simulink model "sinewave"  (R2017a)
settings: Solver=VariableStepAuto  StartTime=0.0  StopTime=100E-6  RelTol=1e-3
libraries: hdlsllib x2
settings Model: Creator=beckmanf  LastModifiedBy=beckmanf
settings OptimizationCC: BlockReduction=off  ConditionallyExecuteInputs=off  DefaultParameterBehavior=Inlined
settings DebuggingCC: AlgebraicLoopMsg=error
settings HardwareCC: ProdBitPerPointer=32  ProdBitPerSizeT=32  ProdBitPerPtrDiffT=32  ProdLargestAtomicFloat=None  ProdIntDivRoundTo=Undefined  ProdEndianess=Unspecified  ProdWordSize=32  ProdHWDeviceType=ASIC/FPGA->ASIC/FPGA  ProdEqTarget=off

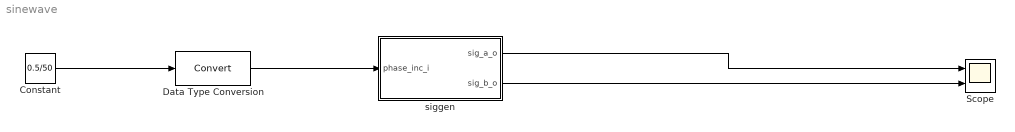
== system sinewave ==
  Constant : Constant  Value=0.5/50  SampleTime=20E-9
  Data Type Conversion : DataTypeConversion
  Scope : Scope  NumInputPorts=2
  siggen : Subsystem
  wires:
  Constant/1 -> Data Type Conversion/1
  Data Type Conversion/1 -> siggen/1(phase_inc_i)
  siggen/1(sig_a_o) -> Scope/1
  siggen/2(sig_b_o) -> Scope/2

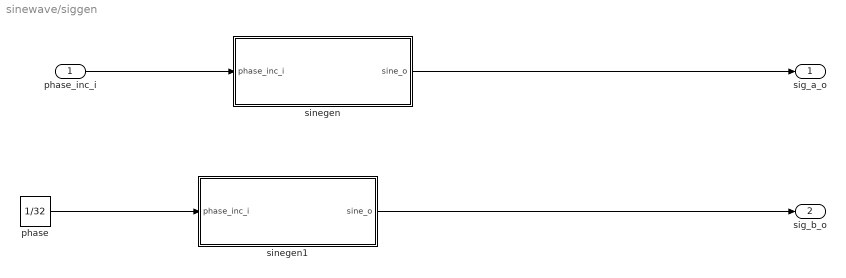
== system sinewave/siggen ==
  phase_inc_i : Inport  OutDataTypeStr=fixdt(0,10,13)
  phase : Constant  Value=1/32  OutDataTypeStr=Inherit: Inherit via back propagation  SampleTime=20E-9
  sinegen : Subsystem
  sinegen1 : Subsystem
  sig_a_o : Outport  OutDataTypeStr=fixdt(1,14,13)
  sig_b_o : Outport  Port=2  OutDataTypeStr=fixdt(1,14,13)
  wires:
  phase_inc_i/1 -> sinegen/1(phase_inc_i)
  phase/1 -> sinegen1/1(phase_inc_i)
  sinegen/1(sine_o) -> sig_a_o/1
  sinegen1/1(sine_o) -> sig_b_o/1

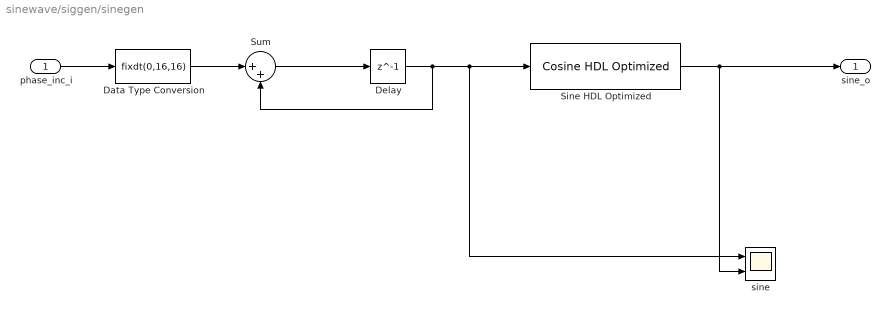
== system sinewave/siggen/sinegen ==
  phase_inc_i : Inport
  Data Type Conversion : DataTypeConversion  OutDataTypeStr=fixdt(0,16,16)
  Delay : Delay  DelayLength=1  InitialCondition=0
  Sine HDL Optimized : hdlsllib/Lookup Tables/Cosine HDL Optimized  OutputFormula=sin(2*pi*u)  NumDataPoints=1024  TableDataTypeStr=fixdt(0,13,13)  SimulateLUTROMDelay=off
      settings: SourceProductName=HDL Coder  SourceProductBaseCode=HD
  Sum : Sum  Inputs=|++  AccumDataTypeStr=fixdt(0,16,16)  OutDataTypeStr=Inherit: Same as accumulator
  sine : Scope  NumInputPorts=2
  sine_o : Outport  OutDataTypeStr=fixdt(1,14,13)
  wires:
  Sine HDL Optimized/1 -> sine/2, sine_o/1
  Delay/1 -> sine/1, Sine HDL Optimized/1, Sum/2
  phase_inc_i/1 -> Data Type Conversion/1
  Data Type Conversion/1 -> Sum/1
  Sum/1 -> Delay/1

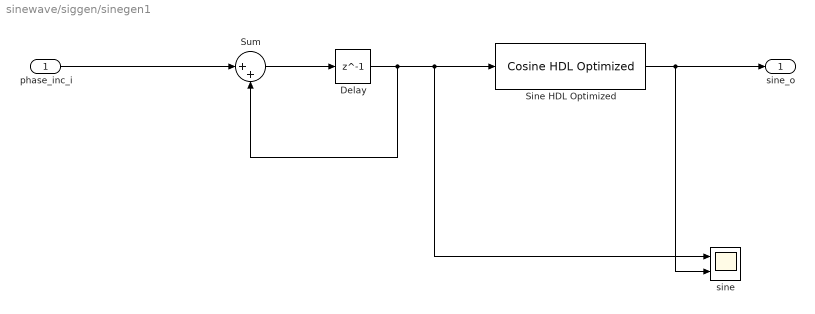
== system sinewave/siggen/sinegen1 ==
  phase_inc_i : Inport  OutDataTypeStr=fixdt(0,16,16)
  Delay : Delay  DelayLength=1  InitialCondition=0
  Sine HDL Optimized : hdlsllib/Lookup Tables/Cosine HDL Optimized  OutputFormula=sin(2*pi*u)  NumDataPoints=128  TableDataTypeStr=fixdt(0,13,13)  SimulateLUTROMDelay=off
      settings: SourceProductName=HDL Coder  SourceProductBaseCode=HD
  Sum : Sum  Inputs=|++  OutDataTypeStr=fixdt(0,16,16)
  sine : Scope  NumInputPorts=2
  sine_o : Outport  OutDataTypeStr=fixdt(1,14,13)
  wires:
  Sine HDL Optimized/1 -> sine/2, sine_o/1
  Delay/1 -> sine/1, Sine HDL Optimized/1, Sum/2
  Sum/1 -> Delay/1
  phase_inc_i/1 -> Sum/1
